simulink model "sl_ztorque"  (Simulink 7.7)
settings: Solver=ode45  StartTime=0.0  StopTime=1  RelTol=1e-3
libraries: roblocks x2
settings Model: Creator=pic  LastModifiedBy=corkep  ExtModeTrigMode=oneshot  ExtModeArmWhenConnect=off
settings DataIOCC: LimitDataPoints=off  SignalLoggingSaveFormat=Dataset  SignalLogging=off  ReturnWorkspaceOutputs=on
settings OptimizationCC: BlockReduction=off  BooleanDataType=off  InitFltsAndDblsToZero=on
settings DebuggingCC: SaveWithParameterizedLinksMsg=none  SignalResolutionControl=TryResolveAllWithWarning  SolverPrmCheckMsg=none  MultiTaskDSMMsg=warning  MultiTaskCondExecSysMsg=none  StrictBusMsg=None
settings HardwareCC: TargetUnknown=on
settings RTWCC: IncludeERTFirstTime=on
settings GRTTargetCC: ModelReferenceCompliant=off  ParMdlRefBuildCompliant=off  CompOptLevelCompliant=off  MatFileLogging=off

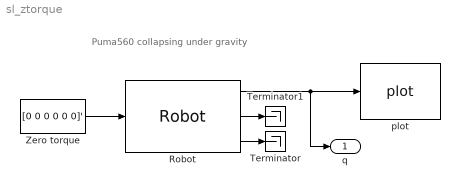
== system sl_ztorque ==
  note: Puma560 collapsing under gravity
  Robot : roblocks/Robot  SystemSampleTime=-1  robot=p560  q0=[0 0 0 0 0 0]
  Terminator : Terminator
  Terminator1 : Terminator
  Zero torque : Constant  Value=[0 0 0 0 0 0]'
  plot : roblocks/plot  SystemSampleTime=-1  robot=p560
  q : Outport
  wires:
  Zero torque/1 -> Robot/1
  Robot/1 -> plot/1, q/1
  Robot/3 -> Terminator/1
  Robot/2 -> Terminator1/1
